simulink model "MdEnCtrlAndBsyChk"  (R2018b)
settings: Solver=FixedStepDiscrete  StartTime=0.0  StopTime=10.0  FixedStep=0.01  RelTol=1e-3
settings Model: Creator=sn2xws  LastModifiedBy=sn2xws
settings DataIOCC: SaveFormat=StructureWithTime
settings OptimizationCC: DefaultParameterBehavior=Inlined  EnhancedBackFolding=on  PassReuseOutputArgsAs=Individual arguments  ZeroExternalMemoryAtStartup=off  ZeroInternalMemoryAtStartup=off  OptimizeBlockOrder=speed  DifferentSizesBufferReuse=on  OptimizationCustomize=off
settings DebuggingCC: ParameterTunabilityLossMsg=error
settings ModelReferenceCC: ModelReferenceNumInstancesAllowed=Single
settings SFSimCC: MATLABDynamicMemAlloc=off
settings RTWCC: SystemTargetFile=autosar.tlc  GenCodeOnly=on  TemplateMakefile=ert_default_tmf  Description=AUTOSAR  GenerateReport=on  IncludeHyperlinkInReport=on  LaunchReport=on  GenerateTraceInfo=on  GenerateTraceReport=on  GenerateTraceReportSl=on  GenerateTraceReportSf=on  GenerateTraceReportEml=on
settings CodeAppCC: ForceParamTrailComments=on  IgnoreCustomStorageClasses=off  OperatorAnnotations=on  SimulinkDataObjDesc=on  SFDataObjDesc=on  InsertBlockDesc=on
settings STFCustomTargetCC: TargetLangStandard=C99 (ISO)  MultiwordLength=256  ParMdlRefBuildCompliant=on  CompOptLevelCompliant=on  IncludeMdlTerminateFcn=off  CombineOutputUpdateFcns=on  SuppressErrorStatus=on  ERTCustomFileBanners=on  SupportNonFinite=off  SupportComplex=off  SupportContinuousTime=off  SupportNonInlinedSFcns=off  RemoveResetFunc=on  MATLABClassNameForMDSCustomization=Simulink.SoftwareTarget.ERTCustomization  AutosarCompliant=on  UseToolchainInfoCompliant=on  LookupTableObjectStructAxisOrder=2,1,3,4,...  LUTObjectStructOrderEvenSpacing=Size,Table,Breakpoints  SystemTargetFile=autosar.tlc
settings ERTTargetCC: TargetLangStandard=C99 (ISO)  ConcurrentExecutionCompliant=off  IncludeMdlTerminateFcn=off  SuppressErrorStatus=on  SupportNonFinite=off  SupportComplex=off  ModelStepFunctionPrototypeControlCompliant=off  CPPClassGenCompliant=off  AutosarCompliant=on  LookupTableObjectStructAxisOrder=2,1,3,4,...  LUTObjectStructOrderEvenSpacing=Size,Table,Breakpoints  InlinedParameterPlacement=NonHierarchical  ERTCustomFileTemplate=example_file_process.tlc

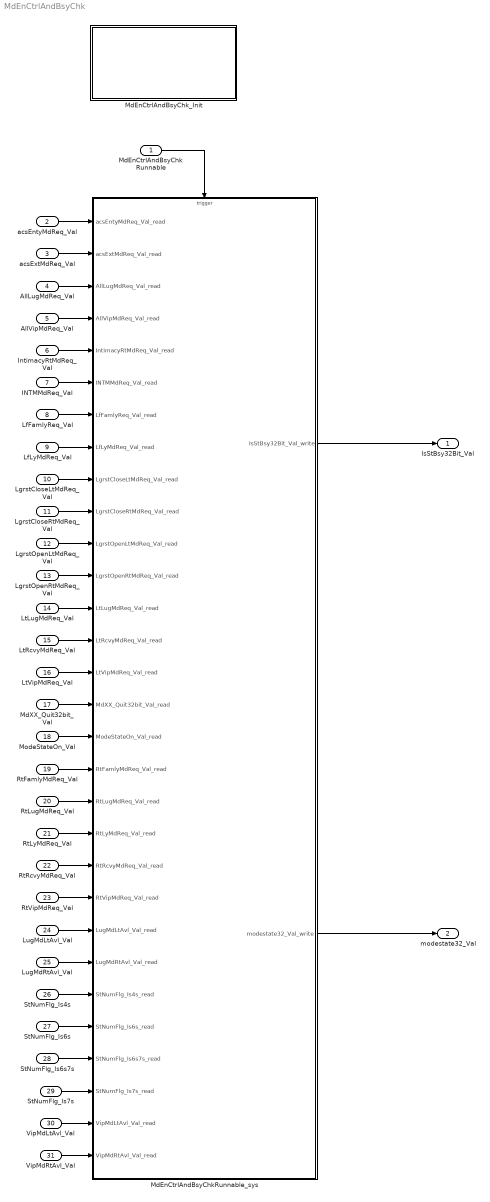
== system MdEnCtrlAndBsyChk ==
  MdEnCtrlAndBsyChkRunnable : Inport  SampleTime=0.01  OutputFunctionCall=on
  acsEntyMdReq_Val : Inport  Port=2  OutDataTypeStr=boolean  PortDimensions=1
  acsExtMdReq_Val : Inport  Port=3  OutDataTypeStr=boolean  PortDimensions=1
  AllLugMdReq_Val : Inport  Port=4  OutDataTypeStr=boolean  PortDimensions=1
  AllVipMdReq_Val : Inport  Port=5  OutDataTypeStr=boolean  PortDimensions=1
  IntimacyRtMdReq_Val : Inport  Port=6  OutDataTypeStr=boolean  PortDimensions=1
  INTMMdReq_Val : Inport  Port=7  OutDataTypeStr=boolean  PortDimensions=1
  LfFamlyReq_Val : Inport  Port=8  OutDataTypeStr=boolean  PortDimensions=1
  LfLyMdReq_Val : Inport  Port=9  OutDataTypeStr=boolean  PortDimensions=1
  LgrstCloseLtMdReq_Val : Inport  Port=10  OutDataTypeStr=boolean  PortDimensions=1
  LgrstCloseRtMdReq_Val : Inport  Port=11  OutDataTypeStr=boolean  PortDimensions=1
  LgrstOpenLtMdReq_Val : Inport  Port=12  OutDataTypeStr=boolean  PortDimensions=1
  LgrstOpenRtMdReq_Val : Inport  Port=13  OutDataTypeStr=boolean  PortDimensions=1
  LtLugMdReq_Val : Inport  Port=14  OutDataTypeStr=boolean  PortDimensions=1
  LtRcvyMdReq_Val : Inport  Port=15  OutDataTypeStr=boolean  PortDimensions=1
  LtVipMdReq_Val : Inport  Port=16  OutDataTypeStr=boolean  PortDimensions=1
  MdXX_Quit32bit_Val : Inport  Port=17  OutDataTypeStr=uint32  PortDimensions=1
  ModeStateOn_Val : Inport  Port=18  OutDataTypeStr=boolean  PortDimensions=1
  RtFamlyMdReq_Val : Inport  Port=19  OutDataTypeStr=boolean  PortDimensions=1
  RtLugMdReq_Val : Inport  Port=20  OutDataTypeStr=boolean  PortDimensions=1
  RtLyMdReq_Val : Inport  Port=21  OutDataTypeStr=boolean  PortDimensions=1
  RtRcvyMdReq_Val : Inport  Port=22  OutDataTypeStr=boolean  PortDimensions=1
  RtVipMdReq_Val : Inport  Port=23  OutDataTypeStr=boolean  PortDimensions=1
  LugMdLtAvl_Val : Inport  Port=24  OutDataTypeStr=boolean  PortDimensions=1
  LugMdRtAvl_Val : Inport  Port=25  OutDataTypeStr=boolean  PortDimensions=1
  StNumFlg_Is4s : Inport  Port=26  OutDataTypeStr=boolean  PortDimensions=1
  StNumFlg_Is6s : Inport  Port=27  OutDataTypeStr=boolean  PortDimensions=1
  StNumFlg_Is6s7s : Inport  Port=28  OutDataTypeStr=boolean  PortDimensions=1
  StNumFlg_Is7s : Inport  Port=29  OutDataTypeStr=boolean  PortDimensions=1
  VipMdLtAvl_Val : Inport  Port=30  OutDataTypeStr=boolean  PortDimensions=1
  VipMdRtAvl_Val : Inport  Port=31  OutDataTypeStr=boolean  PortDimensions=1
  MdEnCtrlAndBsyChkRunnable_sys : Subsystem
  MdEnCtrlAndBsyChk_Init : Subsystem
  IsStBsy32Bit_Val : Outport  OutDataTypeStr=uint32  PortDimensions=1
  modestate32_Val : Outport  Port=2  OutDataTypeStr=uint32  PortDimensions=1
  wires:
  acsEntyMdReq_Val/1 -> MdEnCtrlAndBsyChkRunnable_sys/1(acsEntyMdReq_Val_read)
  acsExtMdReq_Val/1 -> MdEnCtrlAndBsyChkRunnable_sys/2(acsExtMdReq_Val_read)
  AllLugMdReq_Val/1 -> MdEnCtrlAndBsyChkRunnable_sys/3(AllLugMdReq_Val_read)
  AllVipMdReq_Val/1 -> MdEnCtrlAndBsyChkRunnable_sys/4(AllVipMdReq_Val_read)
  IntimacyRtMdReq_Val/1 -> MdEnCtrlAndBsyChkRunnable_sys/5(IntimacyRtMdReq_Val_read)
  INTMMdReq_Val/1 -> MdEnCtrlAndBsyChkRunnable_sys/6(INTMMdReq_Val_read)
  LfFamlyReq_Val/1 -> MdEnCtrlAndBsyChkRunnable_sys/7(LfFamlyReq_Val_read)
  LfLyMdReq_Val/1 -> MdEnCtrlAndBsyChkRunnable_sys/8(LfLyMdReq_Val_read)
  LgrstCloseLtMdReq_Val/1 -> MdEnCtrlAndBsyChkRunnable_sys/9(LgrstCloseLtMdReq_Val_read)
  LgrstCloseRtMdReq_Val/1 -> MdEnCtrlAndBsyChkRunnable_sys/10(LgrstCloseRtMdReq_Val_read)
  LgrstOpenLtMdReq_Val/1 -> MdEnCtrlAndBsyChkRunnable_sys/11(LgrstOpenLtMdReq_Val_read)
  LgrstOpenRtMdReq_Val/1 -> MdEnCtrlAndBsyChkRunnable_sys/12(LgrstOpenRtMdReq_Val_read)
  LtLugMdReq_Val/1 -> MdEnCtrlAndBsyChkRunnable_sys/13(LtLugMdReq_Val_read)
  LtRcvyMdReq_Val/1 -> MdEnCtrlAndBsyChkRunnable_sys/14(LtRcvyMdReq_Val_read)
  LtVipMdReq_Val/1 -> MdEnCtrlAndBsyChkRunnable_sys/15(LtVipMdReq_Val_read)
  MdXX_Quit32bit_Val/1 -> MdEnCtrlAndBsyChkRunnable_sys/16(MdXX_Quit32bit_Val_read)
  ModeStateOn_Val/1 -> MdEnCtrlAndBsyChkRunnable_sys/17(ModeStateOn_Val_read)
  RtFamlyMdReq_Val/1 -> MdEnCtrlAndBsyChkRunnable_sys/18(RtFamlyMdReq_Val_read)
  RtLugMdReq_Val/1 -> MdEnCtrlAndBsyChkRunnable_sys/19(RtLugMdReq_Val_read)
  RtLyMdReq_Val/1 -> MdEnCtrlAndBsyChkRunnable_sys/20(RtLyMdReq_Val_read)
  RtRcvyMdReq_Val/1 -> MdEnCtrlAndBsyChkRunnable_sys/21(RtRcvyMdReq_Val_read)
  RtVipMdReq_Val/1 -> MdEnCtrlAndBsyChkRunnable_sys/22(RtVipMdReq_Val_read)
  MdEnCtrlAndBsyChkRunnable/1 -> MdEnCtrlAndBsyChkRunnable_sys/Trigger
  LugMdLtAvl_Val/1 -> MdEnCtrlAndBsyChkRunnable_sys/23(LugMdLtAvl_Val_read)
  LugMdRtAvl_Val/1 -> MdEnCtrlAndBsyChkRunnable_sys/24(LugMdRtAvl_Val_read)
  StNumFlg_Is4s/1 -> MdEnCtrlAndBsyChkRunnable_sys/25(StNumFlg_Is4s_read)
  StNumFlg_Is6s/1 -> MdEnCtrlAndBsyChkRunnable_sys/26(StNumFlg_Is6s_read)
  StNumFlg_Is6s7s/1 -> MdEnCtrlAndBsyChkRunnable_sys/27(StNumFlg_Is6s7s_read)
  MdEnCtrlAndBsyChkRunnable_sys/1(IsStBsy32Bit_Val_write) -> IsStBsy32Bit_Val/1
  MdEnCtrlAndBsyChkRunnable_sys/2(modestate32_Val_write) -> modestate32_Val/1
  StNumFlg_Is7s/1 -> MdEnCtrlAndBsyChkRunnable_sys/28(StNumFlg_Is7s_read)
  VipMdLtAvl_Val/1 -> MdEnCtrlAndBsyChkRunnable_sys/29(VipMdLtAvl_Val_read)
  VipMdRtAvl_Val/1 -> MdEnCtrlAndBsyChkRunnable_sys/30(VipMdRtAvl_Val_read)

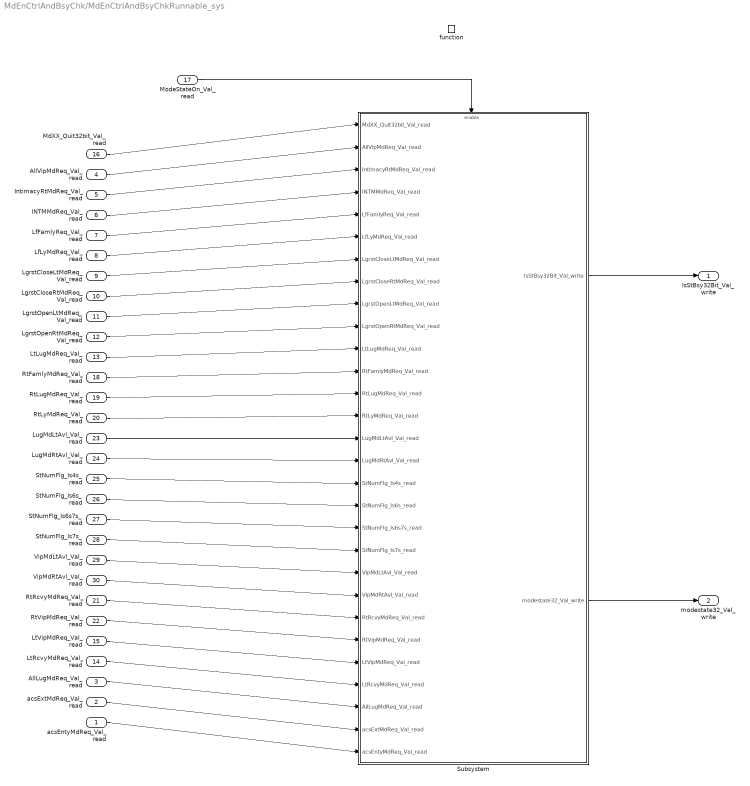
== system MdEnCtrlAndBsyChk/MdEnCtrlAndBsyChkRunnable_sys ==
  acsEntyMdReq_Val_read : Inport
  acsExtMdReq_Val_read : Inport  Port=2
  AllLugMdReq_Val_read : Inport  Port=3
  AllVipMdReq_Val_read : Inport  Port=4
  IntimacyRtMdReq_Val_read : Inport  Port=5
  INTMMdReq_Val_read : Inport  Port=6
  LfFamlyReq_Val_read : Inport  Port=7
  LfLyMdReq_Val_read : Inport  Port=8
  LgrstCloseLtMdReq_Val_read : Inport  Port=9
  LgrstCloseRtMdReq_Val_read : Inport  Port=10
  LgrstOpenLtMdReq_Val_read : Inport  Port=11
  LgrstOpenRtMdReq_Val_read : Inport  Port=12
  LtLugMdReq_Val_read : Inport  Port=13
  LtRcvyMdReq_Val_read : Inport  Port=14
  LtVipMdReq_Val_read : Inport  Port=15
  MdXX_Quit32bit_Val_read : Inport  Port=16
  ModeStateOn_Val_read : Inport  Port=17
  RtFamlyMdReq_Val_read : Inport  Port=18
  RtLugMdReq_Val_read : Inport  Port=19
  RtLyMdReq_Val_read : Inport  Port=20
  RtRcvyMdReq_Val_read : Inport  Port=21
  RtVipMdReq_Val_read : Inport  Port=22
  LugMdLtAvl_Val_read : Inport  Port=23
  LugMdRtAvl_Val_read : Inport  Port=24
  StNumFlg_Is4s_read : Inport  Port=25
  StNumFlg_Is6s_read : Inport  Port=26
  StNumFlg_Is6s7s_read : Inport  Port=27
  StNumFlg_Is7s_read : Inport  Port=28
  VipMdLtAvl_Val_read : Inport  Port=29
  VipMdRtAvl_Val_read : Inport  Port=30
  function : TriggerPort  TriggerType=function-call  VariantControl=(inherit)  SampleTimeType=periodic  SampleTime=-1
  Subsystem : Subsystem
  IsStBsy32Bit_Val_write : Outport
      settings: EnsureOutportIsVirtual=on
  modestate32_Val_write : Outport  Port=2
      settings: EnsureOutportIsVirtual=on
  wires:
  ModeStateOn_Val_read/1 -> Subsystem/Enable
  acsEntyMdReq_Val_read/1 -> Subsystem/29(acsEntyMdReq_Val_read)
  acsExtMdReq_Val_read/1 -> Subsystem/28(acsExtMdReq_Val_read)
  AllLugMdReq_Val_read/1 -> Subsystem/27(AllLugMdReq_Val_read)
  AllVipMdReq_Val_read/1 -> Subsystem/2(AllVipMdReq_Val_read)
  IntimacyRtMdReq_Val_read/1 -> Subsystem/3(IntimacyRtMdReq_Val_read)
  INTMMdReq_Val_read/1 -> Subsystem/4(INTMMdReq_Val_read)
  LfFamlyReq_Val_read/1 -> Subsystem/5(LfFamlyReq_Val_read)
  LfLyMdReq_Val_read/1 -> Subsystem/6(LfLyMdReq_Val_read)
  LgrstCloseLtMdReq_Val_read/1 -> Subsystem/7(LgrstCloseLtMdReq_Val_read)
  LgrstCloseRtMdReq_Val_read/1 -> Subsystem/8(LgrstCloseRtMdReq_Val_read)
  LgrstOpenLtMdReq_Val_read/1 -> Subsystem/9(LgrstOpenLtMdReq_Val_read)
  LgrstOpenRtMdReq_Val_read/1 -> Subsystem/10(LgrstOpenRtMdReq_Val_read)
  LtLugMdReq_Val_read/1 -> Subsystem/11(LtLugMdReq_Val_read)
  LtRcvyMdReq_Val_read/1 -> Subsystem/26(LtRcvyMdReq_Val_read)
  LtVipMdReq_Val_read/1 -> Subsystem/25(LtVipMdReq_Val_read)
  MdXX_Quit32bit_Val_read/1 -> Subsystem/1(MdXX_Quit32bit_Val_read)
  RtFamlyMdReq_Val_read/1 -> Subsystem/12(RtFamlyMdReq_Val_read)
  RtLugMdReq_Val_read/1 -> Subsystem/13(RtLugMdReq_Val_read)
  RtLyMdReq_Val_read/1 -> Subsystem/14(RtLyMdReq_Val_read)
  RtRcvyMdReq_Val_read/1 -> Subsystem/23(RtRcvyMdReq_Val_read)
  RtVipMdReq_Val_read/1 -> Subsystem/24(RtVipMdReq_Val_read)
  LugMdLtAvl_Val_read/1 -> Subsystem/15(LugMdLtAvl_Val_read)
  LugMdRtAvl_Val_read/1 -> Subsystem/16(LugMdRtAvl_Val_read)
  StNumFlg_Is4s_read/1 -> Subsystem/17(StNumFlg_Is4s_read)
  StNumFlg_Is6s_read/1 -> Subsystem/18(StNumFlg_Is6s_read)
  StNumFlg_Is6s7s_read/1 -> Subsystem/19(StNumFlg_Is6s7s_read)
  StNumFlg_Is7s_read/1 -> Subsystem/20(StNumFlg_Is7s_read)
  VipMdLtAvl_Val_read/1 -> Subsystem/21(VipMdLtAvl_Val_read)
  VipMdRtAvl_Val_read/1 -> Subsystem/22(VipMdRtAvl_Val_read)
  Subsystem/2(modestate32_Val_write) -> modestate32_Val_write/1
  Subsystem/1(IsStBsy32Bit_Val_write) -> IsStBsy32Bit_Val_write/1

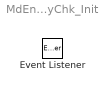
== system MdEnCtrlAndBsyChk/MdEnCtrlAndBsyChk_Init ==
  Event Listener : EventListener  EventName=reset

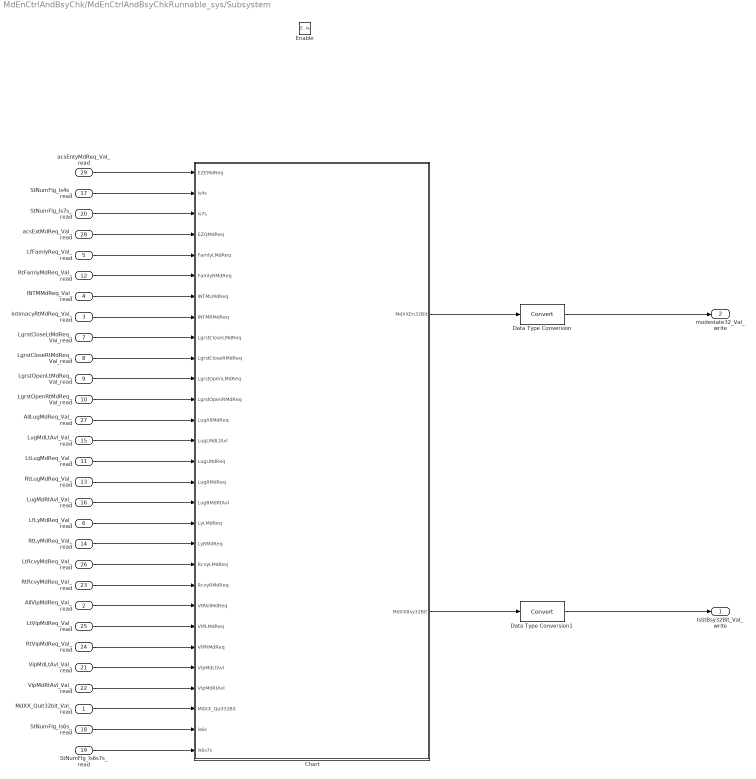
== system MdEnCtrlAndBsyChk/MdEnCtrlAndBsyChkRunnable_sys/Subsystem ==
  MdXX_Quit32bit_Val_read : Inport
  AllVipMdReq_Val_read : Inport  Port=2
  IntimacyRtMdReq_Val_read : Inport  Port=3
  INTMMdReq_Val_read : Inport  Port=4
  LfFamlyReq_Val_read : Inport  Port=5
  LfLyMdReq_Val_read : Inport  Port=6
  LgrstCloseLtMdReq_Val_read : Inport  Port=7
  LgrstCloseRtMdReq_Val_read : Inport  Port=8
  LgrstOpenLtMdReq_Val_read : Inport  Port=9
  LgrstOpenRtMdReq_Val_read : Inport  Port=10
  LtLugMdReq_Val_read : Inport  Port=11
  RtFamlyMdReq_Val_read : Inport  Port=12
  RtLugMdReq_Val_read : Inport  Port=13
  RtLyMdReq_Val_read : Inport  Port=14
  LugMdLtAvl_Val_read : Inport  Port=15
  LugMdRtAvl_Val_read : Inport  Port=16
  StNumFlg_Is4s_read : Inport  Port=17
  StNumFlg_Is6s_read : Inport  Port=18
  StNumFlg_Is6s7s_read : Inport  Port=19
  StNumFlg_Is7s_read : Inport  Port=20
  VipMdLtAvl_Val_read : Inport  Port=21
  VipMdRtAvl_Val_read : Inport  Port=22
  RtRcvyMdReq_Val_read : Inport  Port=23
  RtVipMdReq_Val_read : Inport  Port=24
  LtVipMdReq_Val_read : Inport  Port=25
  LtRcvyMdReq_Val_read : Inport  Port=26
  AllLugMdReq_Val_read : Inport  Port=27
  acsExtMdReq_Val_read : Inport  Port=28
  acsEntyMdReq_Val_read : Inport  Port=29
  Enable : EnablePort  StatesWhenEnabling=reset
  Chart : Stateflow chart  TreatAsAtomicUnit=on
  Data Type Conversion : DataTypeConversion
  Data Type Conversion1 : DataTypeConversion
  IsStBsy32Bit_Val_write : Outport
  modestate32_Val_write : Outport  Port=2
  wires:
  MdXX_Quit32bit_Val_read/1 -> Chart/27(MdXX_Quit32Bit)
  acsEntyMdReq_Val_read/1 -> Chart/1(EZEMdReq)
  acsExtMdReq_Val_read/1 -> Chart/4(EZQMdReq)
  AllLugMdReq_Val_read/1 -> Chart/13(LugAllMdReq)
  IntimacyRtMdReq_Val_read/1 -> Chart/8(INTMRMdReq)
  INTMMdReq_Val_read/1 -> Chart/7(INTMLMdReq)
  LfFamlyReq_Val_read/1 -> Chart/5(FamlyLMdReq)
  LgrstCloseRtMdReq_Val_read/1 -> Chart/10(LgrstCloseRMdReq)
  LgrstCloseLtMdReq_Val_read/1 -> Chart/9(LgrstCloseLMdReq)
  LgrstOpenLtMdReq_Val_read/1 -> Chart/11(LgrstOpenLMdReq)
  LgrstOpenRtMdReq_Val_read/1 -> Chart/12(LgrstOpenRMdReq)
  LtLugMdReq_Val_read/1 -> Chart/15(LugLMdReq)
  LfLyMdReq_Val_read/1 -> Chart/18(LyLMdReq)
  AllVipMdReq_Val_read/1 -> Chart/22(VIPAllMdReq)
  LtVipMdReq_Val_read/1 -> Chart/23(VIPLMdReq)
  RtVipMdReq_Val_read/1 -> Chart/24(VIPRMdReq)
  LtRcvyMdReq_Val_read/1 -> Chart/20(RcvyLMdReq)
  RtRcvyMdReq_Val_read/1 -> Chart/21(RcvyRMdReq)
  RtLugMdReq_Val_read/1 -> Chart/16(LugRMdReq)
  RtLyMdReq_Val_read/1 -> Chart/19(LyRMdReq)
  RtFamlyMdReq_Val_read/1 -> Chart/6(FamlyRMdReq)
  StNumFlg_Is4s_read/1 -> Chart/2(is4s)
  LugMdLtAvl_Val_read/1 -> Chart/14(LugLMdLtAvl)
  LugMdRtAvl_Val_read/1 -> Chart/17(LugRMdRtAvl)
  VipMdLtAvl_Val_read/1 -> Chart/25(VipMdLtAvl)
  VipMdRtAvl_Val_read/1 -> Chart/26(VipMdRtAvl)
  StNumFlg_Is6s_read/1 -> Chart/28(is6s)
  Data Type Conversion/1 -> modestate32_Val_write/1
  Data Type Conversion1/1 -> IsStBsy32Bit_Val_write/1
  Chart/1(MdXXEn32Bit) -> Data Type Conversion/1
  Chart/2(MdXXBsy32Bit) -> Data Type Conversion1/1
  StNumFlg_Is7s_read/1 -> Chart/3(is7s)
  StNumFlg_Is6s7s_read/1 -> Chart/29(is6s7s)

== stateflow chart MdEnCtrlAndBsyChk/MdEnCtrlAndBsyChkRunnable_sys/Subsystem/Chart ==
  settings: executeAtInitialization=1
  state MdEnChk [function]
    (default) -> (junction 1031)
    (junction 1031) -> (junction 1032) [order 1] : [hasChangedTo(EZEMdReq,true)&&((MdXXBsy32Bit&EZEBit)==0)]
    (junction 1031) -> (junction 1033) [order 2]
    (junction 1032) -> (junction 1034) : {
        | MdXXEn32Bit=MdXXEn32Bit|EZEBit;
        | AllMdBsySet();
        | }
    (junction 1034) -> (junction 1033)
    (junction 1033) -> (junction 1035)
    (junction 1035) -> (junction 1036) [order 1] : [hasChangedTo(EZQMdReq,true)&&((MdXXBsy32Bit&EZQBit)==0)]
    (junction 1035) -> (junction 1037) [order 2]
    (junction 1036) -> (junction 1038) : {
        | MdXXEn32Bit=MdXXEn32Bit|EZQBit;
        | AllMdBsySet();
        | }
    (junction 1038) -> (junction 1037)
    (junction 1037) -> (junction 1039)
    (junction 1039) -> (junction 1040) [order 1] : [hasChangedTo(VIPLMdReq,true)&&((MdXXBsy32Bit&VIPLBit)==0)]
    (junction 1039) -> (junction 1041) [order 2]
    (junction 1040) -> (junction 1042) : {
        | MdXXEn32Bit=MdXXEn32Bit|VIPLBit;
        | LftMdBsySet6s7s();
        | LftMdBsySet4s();
        | MdXXBsy32Bit = MdXXBsy32Bit|(is7s<<8);/*LugRBit*/
        | }
    (junction 1042) -> (junction 1041)
    (junction 1041) -> (junction 1043)
    (junction 1043) -> (junction 1044) [order 1] : [hasChangedTo(VIPRMdReq,true)&&((MdXXBsy32Bit&VIPRBit)==0)]
    (junction 1043) -> (junction 1045) [order 2]
    (junction 1044) -> (junction 1046) : {
        | MdXXEn32Bit=MdXXEn32Bit|VIPRBit;
        | RghtMdBsySet6s7s();
        | RghtMdBsySet4s();
        | MdXXBsy32Bit = MdXXBsy32Bit|(is7s<<7);/*LugLBit*/
        | }
    (junction 1046) -> (junction 1045)
    (junction 1045) -> (junction 1047)
    (junction 1047) -> (junction 1048) [order 1] : [hasChangedTo(VIPAllMdReq,true)&&((MdXXBsy32Bit&VIPAllBit)==0)&&(VipMdLtAvl||VipMdRtAvl)]
    (junction 1047) -> (junction 1049) [order 2]
    (junction 1048) -> (junction 1050) : {
        | MdXXEn32Bit=MdXXEn32Bit|(VipMdLtAvl<<9);
        | MdXXEn32Bit=MdXXEn32Bit|(VipMdRtAvl<<11);
        | MdXXEn32Bit=MdXXEn32Bit|VIPAllBit;
        | AllMdBsySet();
        | }
    (junction 1050) -> (junction 1049)
    (junction 1049) -> (junction 1051)
    (junction 1051) -> (junction 1052) [order 1] : [hasChangedTo(RcvyLMdReq,true)&&((MdXXBsy32Bit&RcvyLBit)==0)]
    (junction 1051) -> (junction 1053) [order 2]
    (junction 1052) -> (junction 1054) : {
        | MdXXEn32Bit=MdXXEn32Bit|RcvyLBit;
        | LftMdBsySet6s7s();
        | LftMdBsySet4s();
        | MdXXBsy32Bit = MdXXBsy32Bit|(is7s<<8);/*LugRBit*/
        | }
    (junction 1054) -> (junction 1053)
    (junction 1053) -> (junction 1055)
    (junction 1055) -> (junction 1056) [order 1] : [hasChangedTo(RcvyRMdReq,true)&&((MdXXBsy32Bit&RcvyRBit)==0)]
    (junction 1055) -> (junction 1057) [order 2]
    (junction 1056) -> (junction 1058) : {
        | MdXXEn32Bit=MdXXEn32Bit|RcvyRBit;
        | RghtMdBsySet6s7s();
        | RghtMdBsySet4s();
        | MdXXBsy32Bit = MdXXBsy32Bit|(is7s<<7);/*LugLBit*/
        | }
    (junction 1058) -> (junction 1057)
    (junction 1057) -> (junction 1059)
    (junction 1059) -> (junction 1060) [order 1] : [hasChangedTo(FamlyLMdReq,true)&&((MdXXBsy32Bit&FamlyLBit)==0)]
    (junction 1059) -> (junction 1061) [order 2]
    (junction 1060) -> (junction 1062) : {
        | MdXXEn32Bit=MdXXEn32Bit|FamlyLBit;
        | AllMdBsySet();
        | }
    (junction 1062) -> (junction 1061)
    (junction 1061) -> (junction 1063)
    (junction 1063) -> (junction 1064) [order 1] : [hasChangedTo(FamlyRMdReq,true)&&((MdXXBsy32Bit&FamlyRBit)==0)]
    (junction 1063) -> (junction 1065) [order 2]
    (junction 1064) -> (junction 1066) : {
        | MdXXEn32Bit=MdXXEn32Bit|FamlyRBit;
        | AllMdBsySet();
        | }
    (junction 1066) -> (junction 1065)
    (junction 1065) -> (junction 1067)
    (junction 1067) -> (junction 1068) [order 1] : [hasChangedTo(INTMLMdReq,true)&&((MdXXBsy32Bit&INTMLBit)==0)]
    (junction 1067) -> (junction 1069) [order 2]
    (junction 1068) -> (junction 1070) : {
        | MdXXEn32Bit=MdXXEn32Bit|INTMLBit;
        | AllMdBsySet();
        | }
    (junction 1070) -> (junction 1069)
    (junction 1069) -> (junction 1071)
    (junction 1071) -> (junction 1072) [order 1] : [hasChangedTo(INTMRMdReq,true)&&((MdXXBsy32Bit&INTMRBit)==0)]
    (junction 1071) -> (junction 1073) [order 2]
    (junction 1072) -> (junction 1074) : {
        | MdXXEn32Bit=MdXXEn32Bit|INTMRBit;
        | AllMdBsySet();
        | }
    (junction 1074) -> (junction 1073)
    (junction 1073) -> (junction 1075)
    (junction 1075) -> (junction 1076) [order 1] : [hasChangedTo(LugLMdReq,true)&&((MdXXBsy32Bit&LugLBit)==0)]
    (junction 1075) -> (junction 1077) [order 2]
    (junction 1076) -> (junction 1078) : {
        | MdXXEn32Bit=MdXXEn32Bit|LugLBit;
        | LftMdBsySet6s7s();
        | MdXXBsy32Bit = MdXXBsy32Bit|(is7s<<12);/*RcvyRBit*/
        | MdXXBsy32Bit = MdXXBsy32Bit|(is7s<<11);/*VIPRBit*/
        | }
    (junction 1078) -> (junction 1077)
    (junction 1077) -> (junction 1079)
    (junction 1079) -> (junction 1080) [order 1] : [hasChangedTo(LugRMdReq,true)&&((MdXXBsy32Bit&LugRBit)==0)]
    (junction 1079) -> (junction 1081) [order 2]
    (junction 1080) -> (junction 1082) : {
        | MdXXEn32Bit=MdXXEn32Bit|LugRBit;
        | RghtMdBsySet6s7s();
        | MdXXBsy32Bit = MdXXBsy32Bit|(is7s<<10);/*RcvyLBit*/
        | MdXXBsy32Bit = MdXXBsy32Bit|(is7s<<9);/*VIPLBit*/
        | }
    (junction 1082) -> (junction 1081)
    (junction 1081) -> (junction 1083)
    (junction 1083) -> (junction 1084) [order 1] : [hasChangedTo(LugAllMdReq,true)&&((MdXXBsy32Bit&LugAllBit)==0)&&(LugLMdLtAvl||LugRMdRtAvl)]
    (junction 1083) -> (junction 1085) [order 2]
    (junction 1084) -> (junction 1086) : {
        | MdXXEn32Bit=MdXXEn32Bit|(LugLMdLtAvl<<7);
        | MdXXEn32Bit =MdXXEn32Bit|(LugRMdRtAvl<<8);
        | MdXXEn32Bit=MdXXEn32Bit|LugAllBit;
        | AllMdBsySet();
        | }
    (junction 1086) -> (junction 1085)
    (junction 1085) -> (junction 1087)
    (junction 1087) -> (junction 1088) [order 1] : [is4s&&hasChangedTo(LyLMdReq,true)&&((MdXXBsy32Bit&LyLBit)==0)]
    (junction 1087) -> (junction 1089) [order 2]
    (junction 1088) -> (junction 1090) : {
        | MdXXEn32Bit=MdXXEn32Bit|LyLBit;
        | LftMdBsySet4s();}
    (junction 1090) -> (junction 1089)
    (junction 1089) -> (junction 1091)
    (junction 1091) -> (junction 1092) [order 1] : [is4s&&hasChangedTo(LyRMdReq,true)&&((MdXXBsy32Bit&LyRBit)==0)]
    (junction 1091) -> (junction 1093) [order 2]
    (junction 1092) -> (junction 1094) : {
        | MdXXEn32Bit=MdXXEn32Bit|LyRBit;
        | RghtMdBsySet4s();
        | }
    (junction 1094) -> (junction 1093)
    (junction 1093) -> (junction 1095)
    (junction 1095) -> (junction 1096) [order 1] : [is4s&&hasChangedTo(LgrstOpenLMdReq,true)&&((MdXXBsy32Bit&LgrstOpenLBit)==0)]
    (junction 1095) -> (junction 1097) [order 2]
    (junction 1096) -> (junction 1098) : {
        | MdXXEn32Bit=MdXXEn32Bit|LgrstOpenLBit;
        | LftMdBsySet4s();
        | }
    (junction 1098) -> (junction 1097)
    (junction 1097) -> (junction 1099)
    (junction 1099) -> (junction 1100) [order 1] : [is4s&&hasChangedTo(LgrstOpenRMdReq,true)&&((MdXXBsy32Bit&LgrstOpenRBit)==0)]
    (junction 1099) -> (junction 1101) [order 2]
    (junction 1100) -> (junction 1102) : {
        | MdXXEn32Bit=MdXXEn32Bit|LgrstOpenRBit;
        | RghtMdBsySet4s();
        | }
    (junction 1102) -> (junction 1101)
    (junction 1101) -> (junction 1103)
    (junction 1103) -> (junction 1104) [order 1] : [is4s&&hasChangedTo(LgrstCloseLMdReq,true)&&((MdXXBsy32Bit&LgrstCloseLBit)==0)]
    (junction 1103) -> (junction 1105) [order 2]
    (junction 1104) -> (junction 1106) : {
        | MdXXEn32Bit=MdXXEn32Bit|LgrstCloseLBit;
        | LftMdBsySet4s();
        | }
    (junction 1106) -> (junction 1105)
    (junction 1105) -> (junction 1107)
    (junction 1107) -> (junction 1108) [order 1] : [is4s&&hasChangedTo(LgrstCloseRMdReq,true)&&((MdXXBsy32Bit&LgrstCloseRBit)==0)]
    (junction 1107) -> (junction 1109) [order 2]
    (junction 1108) -> (junction 1110) : {
        | MdXXEn32Bit=MdXXEn32Bit|LgrstCloseRBit;
        | RghtMdBsySet4s();}
    (junction 1110) -> (junction 1109)
    (junction 1109) -> (junction 1111)
  state OnState
    en:MdXXEn32Bit=0;
    en:MdXXBsy32Bit = 0;
    en:MdEnChk();
    du:MdEnClear();
    du:MdBsyClear();
    du:MdEnChk();
  state MdEnClear [function]
    (default) -> (junction 642)
    (junction 642) -> (junction 644) [order 1] : [MdXX_Quit32Bit&EZEBit]
    (junction 642) -> (junction 648) [order 2]
    (junction 644) -> (junction 646) : {
        | MdXXEn32Bit=MdXXEn32Bit&(~EZEBit);
        |
        | }
    (junction 646) -> (junction 648)
    (junction 648) -> (junction 651)
    (junction 651) -> (junction 653) [order 1] : [MdXX_Quit32Bit&EZQBit]
    (junction 651) -> (junction 657) [order 2]
    (junction 653) -> (junction 655) : {
        | MdXXEn32Bit=MdXXEn32Bit&(~EZQBit);
        | }
    (junction 655) -> (junction 657)
    (junction 657) -> (junction 664)
    (junction 664) -> (junction 668) [order 1] : [(MdXX_Quit32Bit&VIPLBit)||((MdXXEn32Bit&VIPAllBit)&&(MdXX_Quit32Bit&VIPAllBit))]
    (junction 664) -> (junction 665) [order 2]
    (junction 668) -> (junction 666) : {
        | MdXXEn32Bit=MdXXEn32Bit&(~VIPLBit);
        | }
    (junction 666) -> (junction 665)
    (junction 665) -> (junction 673)
    (junction 673) -> (junction 677) [order 1] : [(MdXX_Quit32Bit&VIPRBit)||((MdXXEn32Bit&VIPAllBit)&&(MdXX_Quit32Bit&VIPAllBit))]
    (junction 673) -> (junction 674) [order 2]
    (junction 677) -> (junction 675) : {
        | MdXXEn32Bit=MdXXEn32Bit&(~VIPRBit);
        | }
    (junction 675) -> (junction 674)
    (junction 674) -> (junction 682)
    (junction 682) -> (junction 686) [order 1] : [(MdXXEn32Bit&VIPLBit)==0&&(MdXXEn32Bit&VIPRBit)==0]
    (junction 682) -> (junction 683) [order 2]
    (junction 686) -> (junction 684) : {
        | MdXXEn32Bit=MdXXEn32Bit&(~VIPAllBit);
        | }
    (junction 684) -> (junction 683)
    (junction 683) -> (junction 691)
    (junction 691) -> (junction 695) [order 1] : [MdXX_Quit32Bit&RcvyLBit]
    (junction 691) -> (junction 692) [order 2]
    (junction 695) -> (junction 693) : {
        | MdXXEn32Bit=MdXXEn32Bit&(~RcvyLBit);
        | }
    (junction 693) -> (junction 692)
    (junction 692) -> (junction 700)
    (junction 700) -> (junction 704) [order 1] : [MdXX_Quit32Bit&RcvyRBit]
    (junction 700) -> (junction 701) [order 2]
    (junction 704) -> (junction 702) : {
        | MdXXEn32Bit=MdXXEn32Bit&(~RcvyRBit);
        | }
    (junction 702) -> (junction 701)
    (junction 701) -> (junction 709)
    (junction 709) -> (junction 713) [order 1] : [MdXX_Quit32Bit&FamlyLBit]
    (junction 709) -> (junction 710) [order 2]
    (junction 713) -> (junction 711) : {
        | MdXXEn32Bit=MdXXEn32Bit&(~FamlyLBit);
        | }
    (junction 711) -> (junction 710)
    (junction 710) -> (junction 718)
    (junction 718) -> (junction 722) [order 1] : [MdXX_Quit32Bit&FamlyRBit]
    (junction 718) -> (junction 719) [order 2]
    (junction 722) -> (junction 720) : {
        | MdXXEn32Bit=MdXXEn32Bit&(~FamlyRBit);
        | }
    (junction 720) -> (junction 719)
    (junction 719) -> (junction 727)
    (junction 727) -> (junction 731) [order 1] : [MdXX_Quit32Bit&INTMLBit]
    (junction 727) -> (junction 728) [order 2]
    (junction 731) -> (junction 729) : {
        | MdXXEn32Bit=MdXXEn32Bit&(~INTMLBit);
        | }
    (junction 729) -> (junction 728)
    (junction 728) -> (junction 736)
    (junction 736) -> (junction 740) [order 1] : [MdXX_Quit32Bit&INTMRBit]
    (junction 736) -> (junction 737) [order 2]
    (junction 740) -> (junction 738) : {
        | MdXXEn32Bit=MdXXEn32Bit&(~INTMRBit);
        | }
    (junction 738) -> (junction 737)
    (junction 737) -> (junction 751)
    (junction 751) -> (junction 755) [order 1] : [(MdXX_Quit32Bit&LugLBit)||((MdXXEn32Bit&LugAllBit)&&(MdXX_Quit32Bit&LugAllBit))]
    (junction 751) -> (junction 752) [order 2]
    (junction 755) -> (junction 754) : {
        | MdXXEn32Bit=MdXXEn32Bit&(~LugLBit);
        | }
    (junction 754) -> (junction 752)
    (junction 752) -> (junction 760)
    (junction 760) -> (junction 764) [order 1] : [(MdXX_Quit32Bit&LugRBit)||((MdXXEn32Bit&LugAllBit)&&(MdXX_Quit32Bit&LugAllBit))]
    (junction 760) -> (junction 761) [order 2]
    (junction 764) -> (junction 763) : {
        | MdXXEn32Bit=MdXXEn32Bit&(~LugRBit);
        | }
    (junction 763) -> (junction 761)
    (junction 761) -> (junction 769)
    (junction 769) -> (junction 773) [order 1] : [(MdXXEn32Bit&LugLBit)==0&&(MdXXEn32Bit&LugRBit)==0]
    (junction 769) -> (junction 770) [order 2]
    (junction 773) -> (junction 772) : {
        | MdXXEn32Bit=MdXXEn32Bit&(~LugAllBit);
        | }
    (junction 772) -> (junction 770)
    (junction 770) -> (junction 778)
    (junction 778) -> (junction 782) [order 1] : [MdXX_Quit32Bit&LyLBit]
    (junction 778) -> (junction 779) [order 2]
    (junction 782) -> (junction 781) : {
        | MdXXEn32Bit=MdXXEn32Bit&(~LyLBit);
        | }
    (junction 781) -> (junction 779)
    (junction 779) -> (junction 787)
    (junction 787) -> (junction 791) [order 1] : [MdXX_Quit32Bit&LyRBit]
    (junction 787) -> (junction 788) [order 2]
    (junction 791) -> (junction 790) : {
        | MdXXEn32Bit=MdXXEn32Bit&(~LyRBit);
        | }
    (junction 790) -> (junction 788)
    (junction 788) -> (junction 796)
    (junction 796) -> (junction 800) [order 1] : [MdXX_Quit32Bit&LgrstOpenLBit]
    (junction 796) -> (junction 797) [order 2]
    (junction 800) -> (junction 799) : {
        | MdXXEn32Bit=MdXXEn32Bit&(~LgrstOpenLBit);
        | }
    (junction 799) -> (junction 797)
    (junction 797) -> (junction 805)
    (junction 805) -> (junction 809) [order 1] : [MdXX_Quit32Bit&LgrstOpenRBit]
    (junction 805) -> (junction 806) [order 2]
    (junction 809) -> (junction 808) : {
        | MdXXEn32Bit=MdXXEn32Bit&(~LgrstOpenRBit);
        | }
    (junction 808) -> (junction 806)
    (junction 806) -> (junction 814)
    (junction 814) -> (junction 818) [order 1] : [MdXX_Quit32Bit&LgrstCloseLBit]
    (junction 814) -> (junction 815) [order 2]
    (junction 818) -> (junction 817) : {
        | MdXXEn32Bit=MdXXEn32Bit&(~LgrstCloseLBit);
        | }
    (junction 817) -> (junction 815)
    (junction 815) -> (junction 823)
    (junction 823) -> (junction 827) [order 1] : [MdXX_Quit32Bit&LgrstCloseRBit]
    (junction 823) -> (junction 824) [order 2]
    (junction 827) -> (junction 826) : {
        | MdXXEn32Bit=MdXXEn32Bit&(~LgrstCloseRBit);
        | }
    (junction 826) -> (junction 824)
    (junction 824) -> (junction 831)
  state MdBsyClear [function]
    (default) -> (junction 913) : {
        | AllMdBit = EZEBit+EZQBit+VIPAllBit+LugAllBit+INTMLBit+INTMRBit+FamlyLBit+FamlyRBit;
        | LftMdBit6s7s = VIPLBit+RcvyLBit + LugLBit;
        | RghtMdBit6s7s =  VIPRBit+RcvyRBit + LugRBit;
        | LftMdBit4s = VIPLBit+RcvyLBit+LyLBit+LgrstOpenLBit+LgrstCloseLBit;
        | RghtMdBit4s = VIPRBit+RcvyRBit+LyRBit+LgrstOpenRBit+LgrstCloseRBit;
        | }
    (junction 913) -> (junction 915)
    (junction 915) -> (junction 917) [order 1] : [is4s&&((MdXXEn32Bit&LftMdBit4s) == 0)]
    (junction 915) -> (junction 943) [order 2]
    (junction 917) -> (junction 919) : {MdXXBsy32Bit = MdXXBsy32Bit & (~LftMdBit4s);}
    (junction 919) -> (junction 943)
    (junction 943) -> (junction 921)
    (junction 921) -> (junction 923) [order 1] : [is4s && ((MdXXEn32Bit&RghtMdBit4s) == 0)]
    (junction 921) -> (junction 927) [order 2]
    (junction 923) -> (junction 925) : {MdXXBsy32Bit = MdXXBsy32Bit & (~RghtMdBit4s);}
    (junction 925) -> (junction 927)
    (junction 927) -> (junction 935)
    (junction 935) -> (junction 946) [order 1] : [is6s||is7s]
    (junction 946) -> (junction 937) [order 1] : [(MdXXEn32Bit&AllMdBit) == 0]
    (junction 935) -> (junction 948) [order 2]
    (junction 946) -> (junction 950) [order 2]
    (junction 937) -> (junction 953)
    (junction 953) -> (junction 939) [order 1] : [(MdXXEn32Bit &LftMdBit6s7s)==0 &&(MdXXEn32Bit &RghtMdBit6s7s)==0]
    (junction 953) -> (junction 959) [order 2]
    (junction 939) -> (junction 941) : {MdXXBsy32Bit = MdXXBsy32Bit & (~(AllMdBit+LftMdBit6s7s+RghtMdBit6s7s));}
    (junction 959) -> (junction 963) [order 1] : [is6s&&((MdXXEn32Bit &LftMdBit6s7s)==0)]
    (junction 959) -> (junction 967) [order 2]
    (junction 963) -> (junction 965) : {MdXXBsy32Bit = MdXXBsy32Bit &(~LftMdBit6s7s);}
    (junction 967) -> (junction 977) [order 1] : [is7s&&((MdXXEn32Bit &(LftMdBit6s7s+LugRBit))==0)]
    (junction 967) -> (junction 991) [order 2]
    (junction 977) -> (junction 976) : {MdXXBsy32Bit = MdXXBsy32Bit &(~(RcvyLBit+VIPLBit));}
    (junction 976) -> (junction 991)
    (junction 991) -> (junction 974)
    (junction 974) -> (junction 984) [order 1] : [is7s&&((MdXXEn32Bit &(LftMdBit6s7s+RcvyRBit+VIPRBit))==0)]
    (junction 974) -> (junction 979) [order 2]
    (junction 984) -> (junction 988) : {MdXXBsy32Bit = MdXXBsy32Bit &(~(LugLBit));}
    (junction 988) -> (junction 979)
    (junction 965) -> (junction 988)
    (junction 979) -> (junction 986)
    (junction 986) -> (junction 969) [order 1] : [is6s&&((MdXXEn32Bit &RghtMdBit6s7s)==0)]
    (junction 986) -> (junction 995) [order 2]
    (junction 969) -> (junction 971) : {MdXXBsy32Bit = MdXXBsy32Bit &(~RghtMdBit6s7s);}
    (junction 995) -> (junction 997) [order 1] : [is7s&&((MdXXEn32Bit &(RghtMdBit6s7s+LugLBit))==0)]
    (junction 995) -> (junction 1001) [order 2]
    (junction 997) -> (junction 999) : {MdXXBsy32Bit = MdXXBsy32Bit &(~(RcvyRBit+VIPRBit));}
    (junction 999) -> (junction 1001)
    (junction 1001) -> (junction 1004)
    (junction 1004) -> (junction 1006) [order 1] : [is7s&&((MdXXEn32Bit &(RghtMdBit6s7s+RcvyLBit+VIPLBit))==0)]
    (junction 1004) -> (junction 1010) [order 2]
    (junction 1006) -> (junction 1008) : {MdXXBsy32Bit = MdXXBsy32Bit &(~(LugRBit));}
    (junction 950) -> (junction 948)
    (junction 1010) -> (junction 950)
    (junction 1008) -> (junction 1010)
    (junction 971) -> (junction 1008)
    (junction 941) -> (junction 971)
  state AllMdBsySet [function]
    (default) -> (junction 510)
    (junction 510) -> (junction 511) : {
        | MdXXBsy32Bit = MdXXBsy32Bit|(EZEBit+EZQBit+VIPLBit+VIPRBit+VIPAllBit+RcvyLBit+RcvyRBit+LugLBit+LugRBit+LugAllBit+FamlyLBit+FamlyRBit+INTMLBit+INTMRBit);
        | }
  state LftMdBsySet6s7s [function]
    (default) -> (junction 515)
    (junction 515) -> (junction 516) : {
        | MdXXBsy32Bit = MdXXBsy32Bit|(EZEBit+EZQBit+VIPLBit+VIPAllBit+RcvyLBit+LugLBit+LugAllBit+FamlyLBit+FamlyRBit+INTMLBit+INTMRBit);
        | }
    (junction 516) -> (junction 548)
  state RghtMdBsySet6s7s [function]
    (default) -> (junction 529)
    (junction 529) -> (junction 531) : {
        | MdXXBsy32Bit = MdXXBsy32Bit|(EZEBit+EZQBit+VIPRBit+VIPAllBit+RcvyRBit+LugRBit+LugAllBit+FamlyLBit+FamlyRBit+INTMLBit+INTMRBit);
        | }
    (junction 531) -> (junction 552)
  state LftMdBsySet4s [function]
    (default) -> (junction 522)
    (junction 522) -> (junction 524) : {
        | MdXXBsy32Bit = MdXXBsy32Bit|(VIPLBit+RcvyLBit+LyLBit+LgrstOpenLBit+LgrstCloseLBit);
        | }
  state RghtMdBsySet4s [function]
    (default) -> (junction 536)
    (junction 536) -> (junction 537) : {
        | MdXXBsy32Bit = MdXXBsy32Bit|(VIPRBit+RcvyRBit+LyRBit+LgrstOpenRBit+LgrstCloseRBit);
        | }
  (default) -> OnState
  data: EZEMdReq input; is4s input; is7s input; EZQMdReq input; FamlyLMdReq input; FamlyRMdReq input; INTMLMdReq input; INTMRMdReq input; LgrstCloseLMdReq input; LgrstCloseRMdReq input; LgrstOpenLMdReq input; LgrstOpenRMdReq input; LugAllMdReq input; LugLMdLtAvl input; LugLMdReq input; LugRMdReq input; LugRMdRtAvl input; LyLMdReq input; LyRMdReq input; RcvyLMdReq input; RcvyRMdReq input; VIPAllMdReq input; VIPLMdReq input; VIPRMdReq input; VipMdLtAvl input; VipMdRtAvl input; EZEBit constant uint32 =1; EZQBit constant uint32 =8; VIPAllBit constant uint32 =2; LugAllBit constant uint32 =4; MdXX_Quit32Bit input uint32; MdXXEn32Bit output uint32; MdXXBsy32Bit output uint32; VIPLBit constant uint32 =512; VIPRBit constant uint32 =2048; RcvyLBit constant uint32 =1024; RcvyRBit constant uint32 =4096; INTMLBit constant uint32 =16; INTMRBit constant uint32 =524288; FamlyLBit constant uint32 =64; FamlyRBit constant uint32 =32; LugLBit constant uint32 =128; LugRBit constant uint32 =256; LyLBit constant uint32 =8192; LyRBit constant uint32 =16384; LgrstOpenLBit constant uint32 =32768; LgrstOpenRBit constant uint32 =131072; LgrstCloseLBit constant uint32 =65536; LgrstCloseRBit constant uint32 =262144; RghtMdBit6s7s local uint32; is6s input; is6s7s input; AllMdBit local uint32; LftMdBit4s local uint32; LftMdBit6s7s local uint32; RghtMdBit4s local uint32
